simulink model "fftAnalysisSynthesis"  (R2022a)
settings: Solver=FixedStepDiscrete  StartTime=0.0  StopTime=simParams.stopTime  RelTol=1e-3
PostLoadFcn:
  | postLoadCallback
InitFcn:
  | initCallback
StopFcn:
  | stopCallback
values from neighbouring files (symbols this model uses):
  modelParams = createFFTFilters(modelParams)    [createModelParams.m]
libraries: hdlsllib x15, simulink x6, dspsrcs4 x3, dsphdlxfrm2 x2, dspsigops x1
CloseFcn:
  | closeCallback
settings Model: Creator=Ross  LastModifiedBy=Ross_admin
settings SolverCC: AlgebraicLoopSolver=TrustRegion
settings DataIOCC: ReturnWorkspaceOutputs=off
settings OptimizationCC: BlockReduction=off  ConditionallyExecuteInputs=off  DefaultParameterBehavior=Inlined
settings DebuggingCC: ReadBeforeWriteMsg=DisableAll  WriteAfterWriteMsg=DisableAll  WriteAfterReadMsg=DisableAll  AlgebraicLoopMsg=error  MultiTaskDSMMsg=none  SingleTaskRateTransMsg=error  UnconnectedInputMsg=warning  UnconnectedOutputMsg=warning  UnconnectedLineMsg=warning  PregeneratedLibrarySubsystemCodeDiagnostic=none  SFMachineParentedDataDiag=warning  ArithmeticOperatorsInVariantConditions=warning
settings HardwareCC: ProdBitPerPointer=32  ProdBitPerSizeT=32  ProdBitPerPtrDiffT=32  ProdLargestAtomicFloat=None  ProdIntDivRoundTo=Undefined  ProdEndianess=Unspecified  ProdWordSize=32  ProdHWDeviceType=ASIC/FPGA->ASIC/FPGA  TargetBitPerPointer=64  TargetBitPerSizeT=64  TargetBitPerPtrDiffT=64  TargetLongLongMode=on  TargetIntDivRoundTo=Zero  TargetEndianess=LittleEndian  TargetWordSize=64  TargetHWDeviceType=Custom Processor->MATLAB Host Computer  ProdEqTarget=off
settings ModelReferenceCC: UpdateModelReferenceTargets=IfOutOfDate
settings SFSimCC: SFSimEcho=off  SimUseLocalCustomCode=off  CustomCodeUndefinedFunction=UseInterfaceOnly
settings RTWCC: RTWUseLocalCustomCode=off  DLArmComputeVersion=19.05

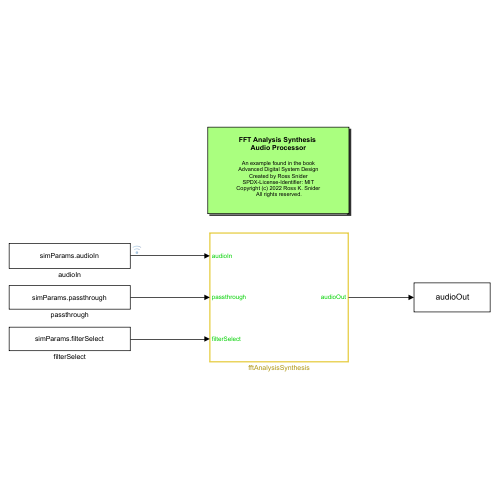
[thumbnail: Simulink's stored preview of the top-level diagram]
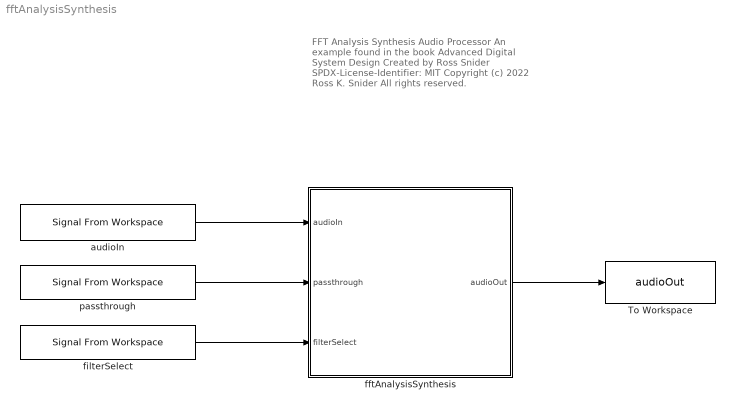
== system fftAnalysisSynthesis ==
  note: FFT Analysis Synthesis
      | Audio Processor
      |
      | An example found in the book
      | Advanced Digital System Design
      | Created by Ross Snider
      | SPDX-License-Identifier: MIT
      | Copyright (c) 2022 Ross K. Snider
      | All rights reserved.
  To Workspace : ToWorkspace  VariableName=audioOut  SampleTime=-1
      settings: Save2DSignal=2-D array (concatenate along first dimension)
  audioIn : dspsrcs4/Signal From Workspace  X=simParams.audioIn  Ts=modelParams.audio.samplePeriod  nsamps=1  OutputAfterFinalValue=Setting to zero  ignoreOrWarnInputAndFrameLengths=off  OutputFrames=off
  fftAnalysisSynthesis : Subsystem  TreatAsAtomicUnit=on
  filterSelect : dspsrcs4/Signal From Workspace  X=simParams.filterSelect  Ts=modelParams.audio.samplePeriod  nsamps=1  OutputAfterFinalValue=Holding final value  ignoreOrWarnInputAndFrameLengths=off  OutputFrames=off
  passthrough : dspsrcs4/Signal From Workspace  X=simParams.passthrough  Ts=modelParams.audio.samplePeriod  nsamps=1  OutputAfterFinalValue=Holding final value  ignoreOrWarnInputAndFrameLengths=off  OutputFrames=off
  wires:
  fftAnalysisSynthesis/1(audioOut) -> To Workspace/1
  audioIn/1 -> fftAnalysisSynthesis/1(audioIn)
  passthrough/1 -> fftAnalysisSynthesis/2(passthrough)
  filterSelect/1 -> fftAnalysisSynthesis/3(filterSelect)

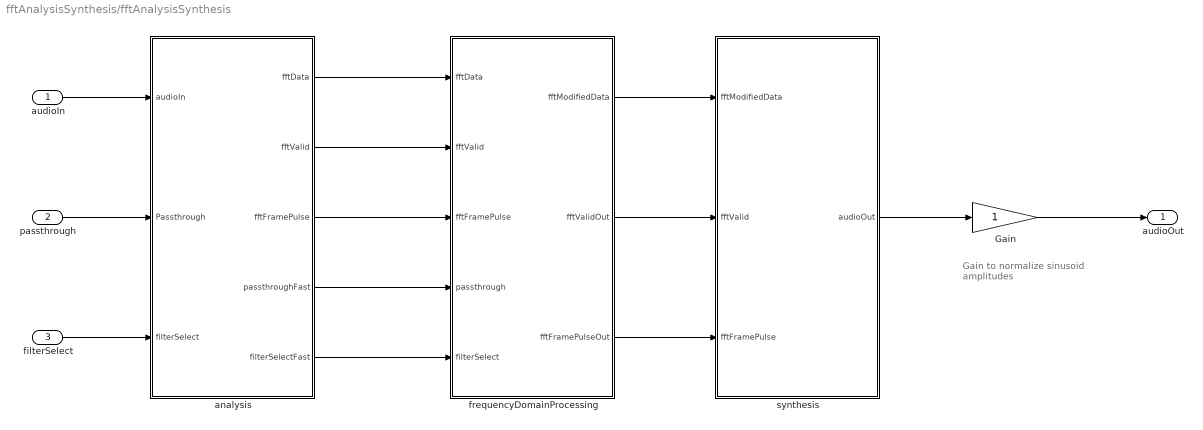
== system fftAnalysisSynthesis/fftAnalysisSynthesis ==
  note: Gain to normalize
      | sinusoid amplitudes
  audioIn : Inport
  passthrough : Inport  Port=2
  filterSelect : Inport  Port=3
  Gain : Gain  OutDataTypeStr=Inherit: Same as input  ParamDataTypeStr=Inherit: Same as input
  analysis : Subsystem
  frequencyDomainProcessing : Subsystem
  synthesis : Subsystem
  audioOut : Outport  VectorParamsAs1DForOutWhenUnconnected=off
  wires:
  audioIn/1 -> analysis/1(audioIn)
  synthesis/1(audioOut) -> Gain/1
  analysis/1(fftData) -> frequencyDomainProcessing/1(fftData)
  analysis/2(fftValid) -> frequencyDomainProcessing/2(fftValid)
  analysis/3(fftFramePulse) -> frequencyDomainProcessing/3(fftFramePulse)
  frequencyDomainProcessing/1(fftModifiedData) -> synthesis/1(fftModifiedData)
  frequencyDomainProcessing/2(fftValidOut) -> synthesis/2(fftValid)
  frequencyDomainProcessing/3(fftFramePulseOut) -> synthesis/3(fftFramePulse)
  analysis/4(passthroughFast) -> frequencyDomainProcessing/4(passthrough)
  passthrough/1 -> analysis/2(Passthrough)
  analysis/5(filterSelectFast) -> frequencyDomainProcessing/5(filterSelect)
  filterSelect/1 -> analysis/3(filterSelect)
  Gain/1 -> audioOut/1

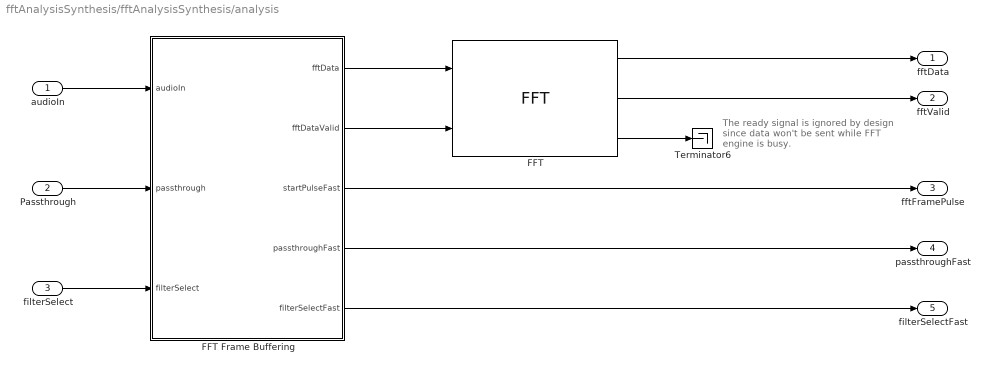
== system fftAnalysisSynthesis/fftAnalysisSynthesis/analysis ==
  note: The ready signal is ignored by design
      | since data won't be sent while FFT
      | engine is busy.
  audioIn : Inport
  Passthrough : Inport  Port=2
  filterSelect : Inport  Port=3
  FFT : dsphdlxfrm2/FFT  FFTLength=modelParams.fft.size  Architecture=Burst Radix 2  ComplexMultiplication=Use 4 multipliers and 2 adders  BitReversedOutput=off  BitReversedInput=off  Normalize=off  SimulateUsing=Code generation  RoundingMethod=Floor  ResetInputPort=off  StartOutputPort=off  EndOutputPort=off
      settings: SourceProductBaseCode=HS
  FFT Frame Buffering : Subsystem
  Terminator6 : Terminator
  fftData : Outport  VectorParamsAs1DForOutWhenUnconnected=off
  fftValid : Outport  Port=2  VectorParamsAs1DForOutWhenUnconnected=off
  fftFramePulse : Outport  Port=3  VectorParamsAs1DForOutWhenUnconnected=off
  passthroughFast : Outport  Port=4
  filterSelectFast : Outport  Port=5
  wires:
  FFT/3 -> Terminator6/1
  FFT Frame Buffering/3(startPulseFast) -> fftFramePulse/1
  audioIn/1 -> FFT Frame Buffering/1(audioIn)
  FFT Frame Buffering/2(fftDataValid) -> FFT/2
  FFT Frame Buffering/1(fftData) -> FFT/1
  FFT/1 -> fftData/1
  FFT/2 -> fftValid/1
  FFT Frame Buffering/4(passthroughFast) -> passthroughFast/1
  Passthrough/1 -> FFT Frame Buffering/2(passthrough)
  filterSelect/1 -> FFT Frame Buffering/3(filterSelect)
  FFT Frame Buffering/5(filterSelectFast) -> filterSelectFast/1

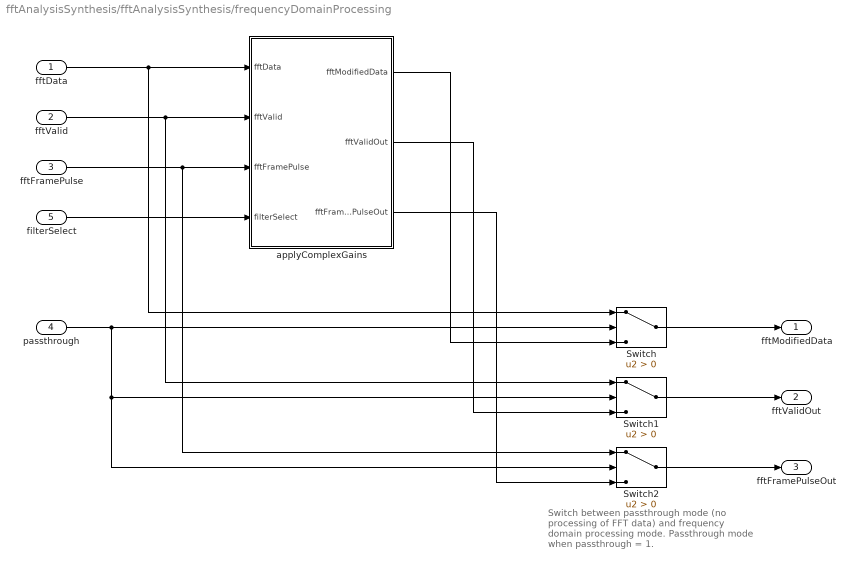
== system fftAnalysisSynthesis/fftAnalysisSynthesis/frequencyDomainProcessing ==
  note: Switch between passthrough mode
      | (no processing of FFT data)
      | and frequency domain processing mode.
      | Passthrough mode when passthrough = 1.
  fftData : Inport
  fftValid : Inport  Port=2
  fftFramePulse : Inport  Port=3
  passthrough : Inport  Port=4
  filterSelect : Inport  Port=5
  Switch : Switch  Criteria=u2 > Threshold  SaturateOnIntegerOverflow=off  InputSameDT=off
  Switch1 : Switch  Criteria=u2 > Threshold  SaturateOnIntegerOverflow=off  InputSameDT=off
  Switch2 : Switch  Criteria=u2 > Threshold  SaturateOnIntegerOverflow=off  InputSameDT=off
  applyComplexGains : Subsystem
  fftModifiedData : Outport  VectorParamsAs1DForOutWhenUnconnected=off
  fftValidOut : Outport  Port=2  VectorParamsAs1DForOutWhenUnconnected=off
  fftFramePulseOut : Outport  Port=3
  wires:
  fftData/1 -> applyComplexGains/1(fftData), Switch/1
  fftValid/1 -> applyComplexGains/2(fftValid), Switch1/1
  applyComplexGains/1(fftModifiedData) -> Switch/3
  applyComplexGains/2(fftValidOut) -> Switch1/3
  fftFramePulse/1 -> applyComplexGains/3(fftFramePulse), Switch2/1
  passthrough/1 -> Switch2/2, Switch1/2, Switch/2
  Switch/1 -> fftModifiedData/1
  applyComplexGains/3(fftFramePulseOut) -> Switch2/3
  Switch1/1 -> fftValidOut/1
  Switch2/1 -> fftFramePulseOut/1
  filterSelect/1 -> applyComplexGains/4(filterSelect)

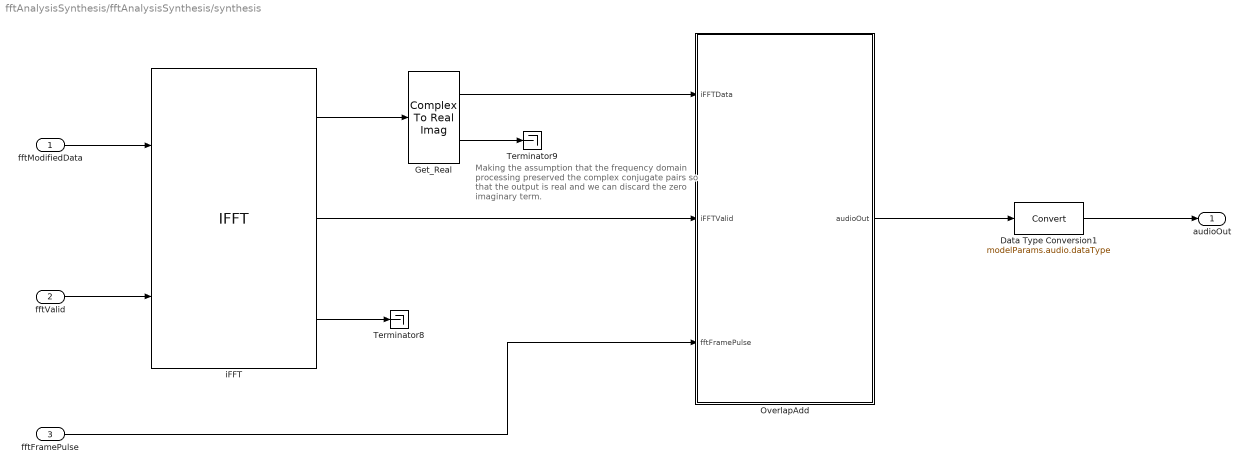
== system fftAnalysisSynthesis/fftAnalysisSynthesis/synthesis ==
  note: Making the assumption that the frequency domain processing preserved the complex conjugate pairs so that the output is real and we can discard the zero imaginary term.
  fftModifiedData : Inport
  fftValid : Inport  Port=2
  fftFramePulse : Inport  Port=3
  Data Type Conversion1 : DataTypeConversion  OutDataTypeStr=modelParams.audio.dataType  SaturateOnIntegerOverflow=off  RndMeth=Floor
  Get_Real : ComplexToRealImag
  OverlapAdd : Subsystem
  Terminator8 : Terminator
  Terminator9 : Terminator
  iFFT : dsphdlxfrm2/IFFT  FFTLength=modelParams.fft.size  Architecture=Burst Radix 2  ComplexMultiplication=Use 4 multipliers and 2 adders  BitReversedOutput=off  BitReversedInput=off  Normalize=on  SimulateUsing=Code generation  RoundingMethod=Floor  ResetInputPort=off  StartOutputPort=off  EndOutputPort=off
      settings: SourceProductBaseCode=HS
  audioOut : Outport  VectorParamsAs1DForOutWhenUnconnected=off
  wires:
  iFFT/3 -> Terminator8/1
  iFFT/2 -> OverlapAdd/2(iFFTValid)
  Get_Real/1 -> OverlapAdd/1(iFFTData)
  fftModifiedData/1 -> iFFT/1
  Data Type Conversion1/1 -> audioOut/1
  iFFT/1 -> Get_Real/1
  Get_Real/2 -> Terminator9/1
  fftValid/1 -> iFFT/2
  fftFramePulse/1 -> OverlapAdd/3(fftFramePulse)
  OverlapAdd/1(audioOut) -> Data Type Conversion1/1

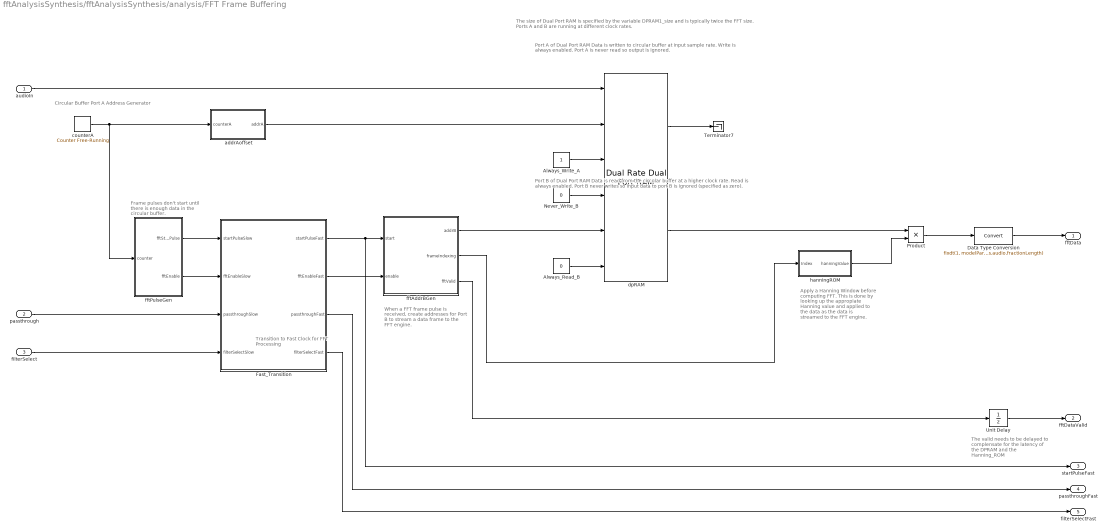
== system fftAnalysisSynthesis/fftAnalysisSynthesis/analysis/FFT Frame Buffering ==
  note: The valid needs to be delayed
      | to complensate for the latency
      | of the DPRAM and the
      | Hanning_ROM
  note: When a FFT frame pulse
      | is received, create addresses for
      | Port B to stream a data frame
      | to the FFT engine.
  note: Apply a Hanning Window
      | before computing FFT.  This
      | is done by looking up the
      | appropiate Hanning value
      | and applied to the data as the
      | data is streamed to the
      | FFT engine.
  note: Frame pulses don't start
      | until there is enough data
      | in the circular buffer.
  note: The size of Dual Port RAM is specified by the variable DPRAM1_size
      | and is typically twice the FFT size.  Ports A and B are running at different clock rates.
  note: Circular Buffer
      | Port A Address Generator
  note: Port A of Dual Port RAM
      |
      | Data is written to circular buffer at input sample rate.
      | Write is always enabled.  Port A is never read so output is ignored.
  note: Transition to
      | Fast Clock
      | for FFT Processing
  note: Port B of Dual Port RAM
      |
      | Data is read from the circular buffer at a higher clock rate.
      | Read is always enabled.  Port B never writes so input data to port B
      | is ignored (specified as zero).
  audioIn : Inport
  passthrough : Inport  Port=2
  filterSelect : Inport  Port=3
  Always_Read_B : Constant  Value=0  OutDataTypeStr=boolean  SampleTime=modelParams.audio.samplePeriod/modelParams.system.upsample_Factor
  Always_Write_A : Constant  OutDataTypeStr=boolean  SampleTime=modelParams.audio.samplePeriod
  Data Type Conversion : DataTypeConversion  OutDataTypeStr=fixdt(1, modelParams.audio.wordLength, modelParams.audio.fractionLength)  SaturateOnIntegerOverflow=off  RndMeth=Floor
  Fast_Transition : Subsystem
  Never_Write_B : Constant  Value=0  OutDataTypeStr=modelParams.audio.dataType  SampleTime=modelParams.audio.samplePeriod/modelParams.system.upsample_Factor
  Product : Product
  Terminator7 : Terminator
  Unit Delay : UnitDelay  SampleTime=-1  HasFrameUpgradeWarning=on
  addrAoffset : Subsystem
  counterA : simulink/Sources/Counter Free-Running  NumBits=modelParams.dpram1.address_size  tsamp=modelParams.audio.samplePeriod
  dpRAM : hdlsllib/HDL RAMs/Dual Rate Dual Port RAM  ram_size=modelParams.dpram1.address_size
      settings: SourceProductBaseCode=SL
  fftAddrBGen : Subsystem
  fftPulseGen : Subsystem
  hanningROM : Subsystem
  fftData : Outport  VectorParamsAs1DForOutWhenUnconnected=off
  fftDataValid : Outport  Port=2  VectorParamsAs1DForOutWhenUnconnected=off
  startPulseFast : Outport  Port=3  VectorParamsAs1DForOutWhenUnconnected=off
  passthroughFast : Outport  Port=4
  filterSelectFast : Outport  Port=5
  wires:
  Always_Write_A/1 -> dpRAM/3
  Never_Write_B/1 -> dpRAM/4
  Always_Read_B/1 -> dpRAM/6
  dpRAM/1 -> Terminator7/1
  fftAddrBGen/3(fftValid) -> Unit Delay/1
  fftAddrBGen/1(addrB) -> dpRAM/5
  counterA/1 -> addrAoffset/1(counterA), fftPulseGen/1(counter)
  audioIn/1 -> dpRAM/1
  addrAoffset/1(addrA) -> dpRAM/2
  fftAddrBGen/2(frameIndexing) -> hanningROM/1(Index)
  Product/1 -> Data Type Conversion/1
  dpRAM/2 -> Product/1
  hanningROM/1(hanningValue) -> Product/2
  Data Type Conversion/1 -> fftData/1
  Fast_Transition/1(startPulseFast) -> startPulseFast/1, fftAddrBGen/1(start)
  fftPulseGen/1(fftStartPulse) -> Fast_Transition/1(startPulseSlow)
  fftPulseGen/2(fftEnable) -> Fast_Transition/2(fftEnableSlow)
  Fast_Transition/2(fftEnableFast) -> fftAddrBGen/2(enable)
  Unit Delay/1 -> fftDataValid/1
  passthrough/1 -> Fast_Transition/3(passthroughSlow)
  Fast_Transition/3(passthroughFast) -> passthroughFast/1
  filterSelect/1 -> Fast_Transition/4(filterSelectSlow)
  Fast_Transition/4(filterSelectFast) -> filterSelectFast/1

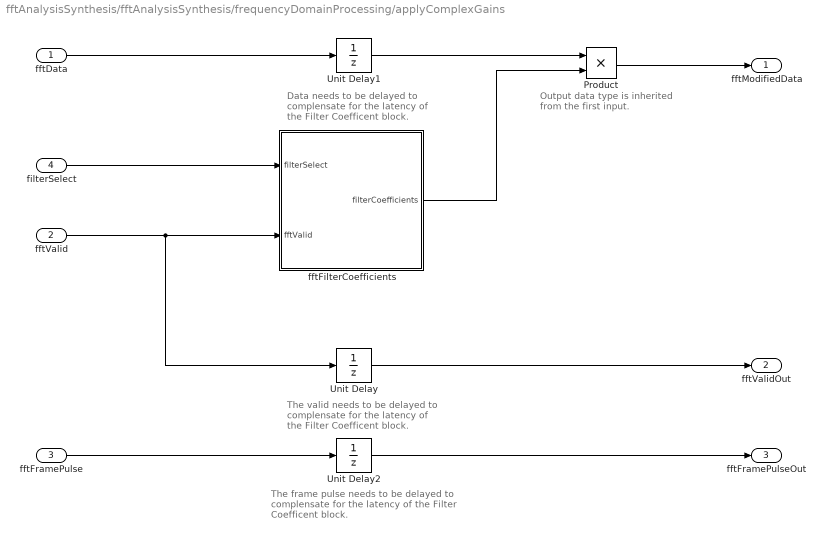
== system fftAnalysisSynthesis/fftAnalysisSynthesis/frequencyDomainProcessing/applyComplexGains ==
  note: Output data type is inherited
      | from the first input.
  note: The frame pulse needs to be delayed
      | to complensate for the latency
      | of the Filter Coefficent block.
  note: The valid needs to be delayed
      | to complensate for the latency
      | of the Filter Coefficent block.
  note: Data needs to be delayed
      | to complensate for the latency
      | of the Filter Coefficent block.
  fftData : Inport
  fftValid : Inport  Port=2
  fftFramePulse : Inport  Port=3
  filterSelect : Inport  Port=4
  Product : Product  OutDataTypeStr=Inherit: Same as first input
  Unit Delay : UnitDelay  SampleTime=-1  HasFrameUpgradeWarning=on
  Unit Delay1 : UnitDelay  SampleTime=-1  HasFrameUpgradeWarning=on
  Unit Delay2 : UnitDelay  SampleTime=-1  HasFrameUpgradeWarning=on
  fftFilterCoefficients : Subsystem
  fftModifiedData : Outport
  fftValidOut : Outport  Port=2
  fftFramePulseOut : Outport  Port=3
  wires:
  fftValid/1 -> Unit Delay/1, fftFilterCoefficients/2(fftValid)
  fftData/1 -> Unit Delay1/1
  fftFramePulse/1 -> Unit Delay2/1
  Unit Delay2/1 -> fftFramePulseOut/1
  filterSelect/1 -> fftFilterCoefficients/1(filterSelect)
  fftFilterCoefficients/1(filterCoefficients) -> Product/2
  Product/1 -> fftModifiedData/1
  Unit Delay/1 -> fftValidOut/1
  Unit Delay1/1 -> Product/1

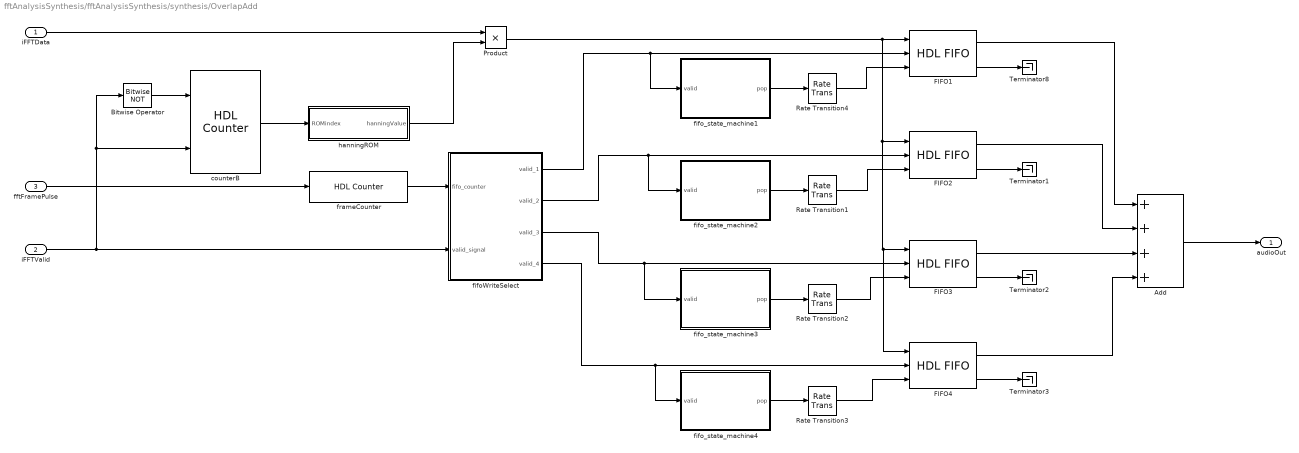
== system fftAnalysisSynthesis/fftAnalysisSynthesis/synthesis/OverlapAdd ==
  iFFTData : Inport
  iFFTValid : Inport  Port=2
  fftFramePulse : Inport  Port=3
  Add : Sum  Inputs=4
  Bitwise Operator : simulink/Logic and Bit Operations/Bitwise Operator  logicop=NOT  UseBitMask=off  BitMask=bin2dec('11011001')  BitMaskRealWorld=Stored Integer
  FIFO{1..4} (4 alike) : hdlsllib/HDL RAMs/HDL FIFO  fifo_size=modelParams.fft.size  mode=Classic  ratio=modelParams.system.upsample_Factor  push_msg=Warning  pop_msg=Warning  show_empty=off  show_full=on  show_num=off  LabelModeActiveChoice_Mode=Classic  rst_port=off
      settings: SourceProductBaseCode=SL
  Product : Product  OutDataTypeStr=Inherit: Same as first input
  Rate Transition{1..4} (4 alike) : RateTransition  OutPortSampleTimeOpt=Multiple of input port sample time  OutPortSampleTimeMultiple=modelParams.system.upsample_Factor
  Terminator{1..3,8} (4 alike) : Terminator
  counterB : hdlsllib/Sources/HDL Counter  CountType=Count limited  CountInit=0  CountStep=1  CountMax=modelParams.fft.size  CountFromType=Initial value  CountFrom=0  CountResetPort=on  CountLoadPort=off  CountEnbPort=on  CountDirPort=off  CountHitOutputPort=off  CountDataType=Unsigned  CountWordLen=modelParams.dpram1.address_size  CountFracLen=0  CountSampTime=1
  fifoWriteSelect : MATLAB Function  TreatAsAtomicUnit=on
  fifo_state_machine1 : MATLAB Function  TreatAsAtomicUnit=on
  fifo_state_machine2 : MATLAB Function  TreatAsAtomicUnit=on
  fifo_state_machine3 : MATLAB Function  TreatAsAtomicUnit=on
  fifo_state_machine4 : MATLAB Function  TreatAsAtomicUnit=on
  frameCounter : hdlsllib/Sources/HDL Counter  CountType=Free running  CountInit=2  CountStep=1  CountMax=1024  CountFromType=Initial value  CountFrom=2  CountResetPort=off  CountLoadPort=off  CountEnbPort=on  CountDirPort=off  CountHitOutputPort=off  CountDataType=Unsigned  CountWordLen=2  CountFracLen=0  CountSampTime=1
  hanningROM : Subsystem
  audioOut : Outport  VectorParamsAs1DForOutWhenUnconnected=off
  wires:
  FIFO1/1 -> Add/1
  FIFO3/1 -> Add/3
  fftFramePulse/1 -> frameCounter/1
  FIFO2/1 -> Add/2
  fifoWriteSelect/3(valid_3) -> fifo_state_machine3/1(valid), FIFO3/2
  fifoWriteSelect/4(valid_4) -> fifo_state_machine4/1(valid), FIFO4/2
  FIFO4/1 -> Add/4
  fifoWriteSelect/1(valid_1) -> fifo_state_machine1/1(valid), FIFO1/2
  fifoWriteSelect/2(valid_2) -> fifo_state_machine2/1(valid), FIFO2/2
  Add/1 -> audioOut/1
  frameCounter/1 -> fifoWriteSelect/1(fifo_counter)
  FIFO4/2 -> Terminator3/1
  FIFO2/2 -> Terminator1/1
  FIFO3/2 -> Terminator2/1
  Bitwise Operator/1 -> counterB/1
  iFFTValid/1 -> counterB/2, Bitwise Operator/1, fifoWriteSelect/2(valid_signal)
  iFFTData/1 -> Product/1
  hanningROM/1(hanningValue) -> Product/2
  counterB/1 -> hanningROM/1(ROMindex)
  fifo_state_machine1/1(pop) -> Rate Transition4/1
  Rate Transition4/1 -> FIFO1/3
  FIFO1/2 -> Terminator8/1
  fifo_state_machine2/1(pop) -> Rate Transition1/1
  Rate Transition1/1 -> FIFO2/3
  fifo_state_machine3/1(pop) -> Rate Transition2/1
  Rate Transition2/1 -> FIFO3/3
  fifo_state_machine4/1(pop) -> Rate Transition3/1
  Rate Transition3/1 -> FIFO4/3
  Product/1 -> FIFO4/1, FIFO3/1, FIFO2/1, FIFO1/1

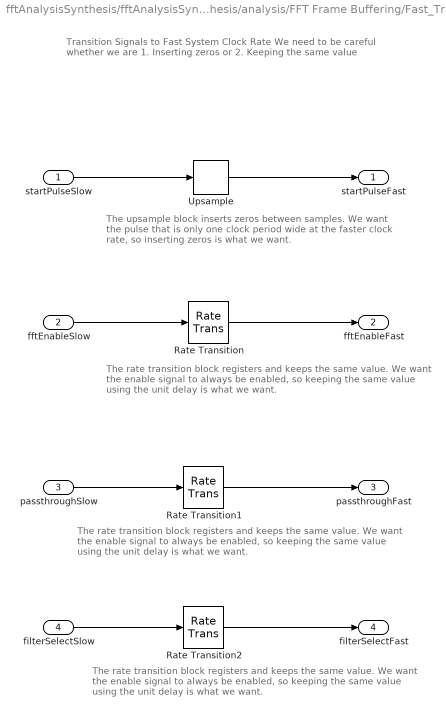
== system fftAnalysisSynthesis/fftAnalysisSynthesis/analysis/FFT Frame Buffering/Fast_Transition ==
  note: The upsample block inserts zeros between samples.
      | We want the pulse that is only one clock period wide at the
      | faster clock rate, so inserting zeros is what we want.
  note: The rate transition block registers and keeps the same
      | value. We want the enable signal to always be enabled,
      | so keeping the same value using the unit delay is what we want.
  note: The rate transition block registers and keeps the same
      | value. We want the enable signal to always be enabled,
      | so keeping the same value using the unit delay is what we want.
  note: The rate transition block registers and keeps the same
      | value. We want the enable signal to always be enabled,
      | so keeping the same value using the unit delay is what we want.
  note: Transition Signals to Fast System Clock Rate
      | We need to be careful whether we are
      | 1. Inserting zeros
      | or
      | 2. Keeping the same value
  startPulseSlow : Inport
  fftEnableSlow : Inport  Port=2
  passthroughSlow : Inport  Port=3
  filterSelectSlow : Inport  Port=4
  Rate Transition : RateTransition  OutPortSampleTimeOpt=Multiple of input port sample time  OutPortSampleTimeMultiple=1/modelParams.system.upsample_Factor
  Rate Transition1 : RateTransition  OutPortSampleTimeOpt=Multiple of input port sample time  OutPortSampleTimeMultiple=1/modelParams.system.upsample_Factor
  Rate Transition2 : RateTransition  InitialCondition=3  OutPortSampleTimeOpt=Multiple of input port sample time  OutPortSampleTimeMultiple=1/modelParams.system.upsample_Factor
  Upsample : dspsigops/Upsample  N=modelParams.system.upsample_Factor  phase=0  RateOptions=Allow multirate processing  ic=0  mode=Unused parameter value
  startPulseFast : Outport
  fftEnableFast : Outport  Port=2
  passthroughFast : Outport  Port=3
  filterSelectFast : Outport  Port=4
  wires:
  startPulseSlow/1 -> Upsample/1
  Rate Transition/1 -> fftEnableFast/1
  fftEnableSlow/1 -> Rate Transition/1
  Upsample/1 -> startPulseFast/1
  passthroughSlow/1 -> Rate Transition1/1
  Rate Transition1/1 -> passthroughFast/1
  filterSelectSlow/1 -> Rate Transition2/1
  Rate Transition2/1 -> filterSelectFast/1

== system fftAnalysisSynthesis/fftAnalysisSynthesis/analysis/FFT Frame Buffering/addrAoffset ==
  note: Adding 1 to counter since the read pointer (addr_B) can catch the write pointer (addr_A)
      | if SysRate_Upsample_Factor is large enough and Simulink will throw an error.
      | It would be nice if the HDL Coder allowed a read-before-write option when
      | the addresses are identical, which some memories support.
  counterA : Inport
  Add : Sum  OutDataTypeStr=fixdt(0,modelParams.dpram1.address_size,0)
  writeOffset : Constant  OutDataTypeStr=fixdt(0,modelParams.dpram1.address_size,0)  SampleTime=modelParams.audio.samplePeriod
  addrA : Outport  VectorParamsAs1DForOutWhenUnconnected=off
  wires:
  writeOffset/1 -> Add/2
  Add/1 -> addrA/1
  counterA/1 -> Add/1

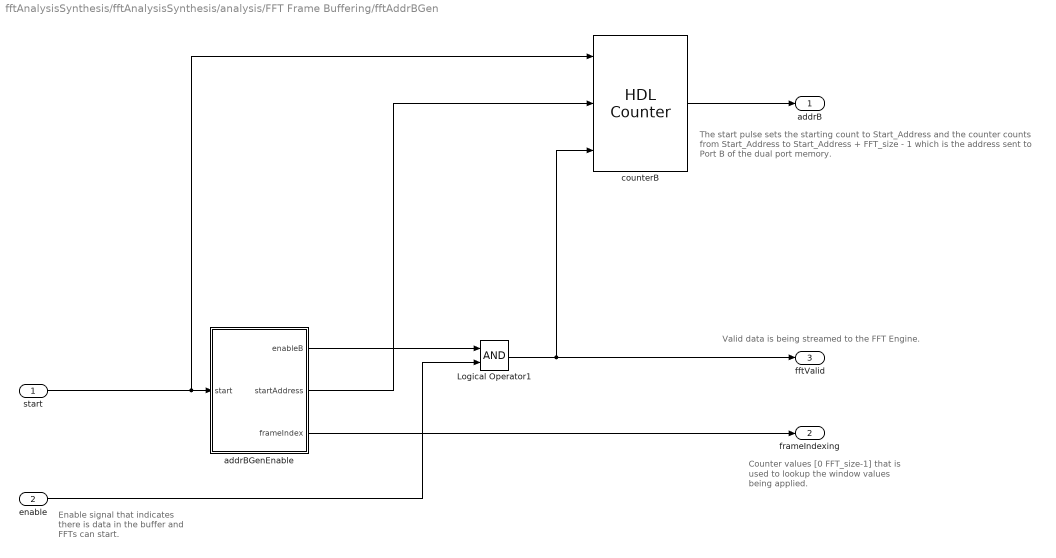
== system fftAnalysisSynthesis/fftAnalysisSynthesis/analysis/FFT Frame Buffering/fftAddrBGen ==
  note: Counter values [0 FFT_size-1] that
      | is used to lookup the window values
      | being applied.
  note: Valid data is being streamed to the FFT Engine.
  note: Enable signal that indicates
      | there is data in the buffer
      | and FFTs can start.
  note: The start pulse sets the starting count to Start_Address
      |  and the counter counts from Start_Address to Start_Address + FFT_size - 1
      | which is the address sent to Port B of the dual port memory.
  start : Inport
  enable : Inport  Port=2
  Logical Operator1 : Logic  AllPortsSameDT=off  OutDataTypeStr=boolean
  addrBGenEnable : Subsystem
  counterB : hdlsllib/Sources/HDL Counter  CountType=Free running  CountInit=modelParams.dpram1.init  CountStep=1  CountMax=1024  CountFromType=Initial value  CountFrom=modelParams.dpram1.init  CountResetPort=off  CountLoadPort=on  CountEnbPort=on  CountDirPort=off  CountHitOutputPort=off  CountDataType=Unsigned  CountWordLen=modelParams.dpram1.address_size  CountFracLen=0  CountSampTime=1
  addrB : Outport  VectorParamsAs1DForOutWhenUnconnected=off
  frameIndexing : Outport  Port=2  VectorParamsAs1DForOutWhenUnconnected=off
  fftValid : Outport  Port=3  VectorParamsAs1DForOutWhenUnconnected=off
  wires:
  counterB/1 -> addrB/1
  start/1 -> counterB/1, addrBGenEnable/1(start)
  addrBGenEnable/1(enableB) -> Logical Operator1/1
  addrBGenEnable/2(startAddress) -> counterB/2
  enable/1 -> Logical Operator1/2
  addrBGenEnable/3(frameIndex) -> frameIndexing/1
  Logical Operator1/1 -> counterB/3, fftValid/1

== system fftAnalysisSynthesis/fftAnalysisSynthesis/analysis/FFT Frame Buffering/fftPulseGen ==
  note: Don't send out FFT frame start pulses
      | until circular buffer has filled.
  counter : Inport
  fftFramePulseGen : Subsystem
  waitForData : Subsystem
  fftStartPulse : Outport  VectorParamsAs1DForOutWhenUnconnected=off
  fftEnable : Outport  Port=2  VectorParamsAs1DForOutWhenUnconnected=off
  wires:
  counter/1 -> fftFramePulseGen/1("counterValue ")
  waitForData/1(fftFramePulse) -> fftStartPulse/1
  waitForData/2(enableFFTframes) -> fftEnable/1
  fftFramePulseGen/1(framePulse) -> waitForData/1(framePulse)

== system fftAnalysisSynthesis/fftAnalysisSynthesis/analysis/FFT Frame Buffering/hanningROM ==
  Index : Inport
  Lookup Table : Lookup_n-D  NumberOfTableDimensions=1  BreakpointsForDimension1=[0:modelParams.fft.size-1]  IndexSearchMethod=Evenly spaced points  Table=hanning(modelParams.fft.size)  InterpMethod=Flat  ExtrapMethod=Clip  DiagnosticForOutOfRangeInput=Warning  UseLastTableValue=on  OutDataTypeStr=fixdt(1,24,23)  RndMeth=Simplest
  Unit Delay : UnitDelay  SampleTime=-1  HasFrameUpgradeWarning=on
  hanningValue : Outport  VectorParamsAs1DForOutWhenUnconnected=off
  wires:
  Unit Delay/1 -> hanningValue/1
  Index/1 -> Lookup Table/1
  Lookup Table/1 -> Unit Delay/1

== system fftAnalysisSynthesis/fftAnalysisSynthesis/frequencyDomainProcessing/applyComplexGains/fftFilterCoefficients ==
  filterSelect : Inport
  fftValid : Inport  Port=2
  fftROMindexing : Subsystem
  filterChoice : Subsystem
  filterCoefficients : Outport
  wires:
  fftROMindexing/1(ROMindex) -> filterChoice/2(ROMindex)
  fftValid/1 -> fftROMindexing/1(fftValid)
  filterSelect/1 -> filterChoice/1(filterSelect)
  filterChoice/1(filterCoefficients) -> filterCoefficients/1

== system fftAnalysisSynthesis/fftAnalysisSynthesis/synthesis/OverlapAdd/hanningROM ==
  ROMindex : Inport
  Bit Slice : hdlsllib/Logic and Bit Operations/Bit Slice  lidx=modelParams.fft.Nbits - 1  ridx=0
      settings: SourceProductBaseCode=SL
  Lookup Table : Lookup_n-D  NumberOfTableDimensions=1  BreakpointsForDimension1=[0:modelParams.fft.size-1]  IndexSearchMethod=Evenly spaced points  Table=hanning(modelParams.fft.size)  InterpMethod=Flat  ExtrapMethod=Clip  DiagnosticForOutOfRangeInput=Error  UseLastTableValue=on  OutDataTypeStr=fixdt(1,24,22)  RndMeth=Simplest
  Unit Delay : UnitDelay  SampleTime=-1  HasFrameUpgradeWarning=on
  hanningValue : Outport  VectorParamsAs1DForOutWhenUnconnected=off
  wires:
  Unit Delay/1 -> hanningValue/1
  ROMindex/1 -> Bit Slice/1
  Lookup Table/1 -> Unit Delay/1
  Bit Slice/1 -> Lookup Table/1

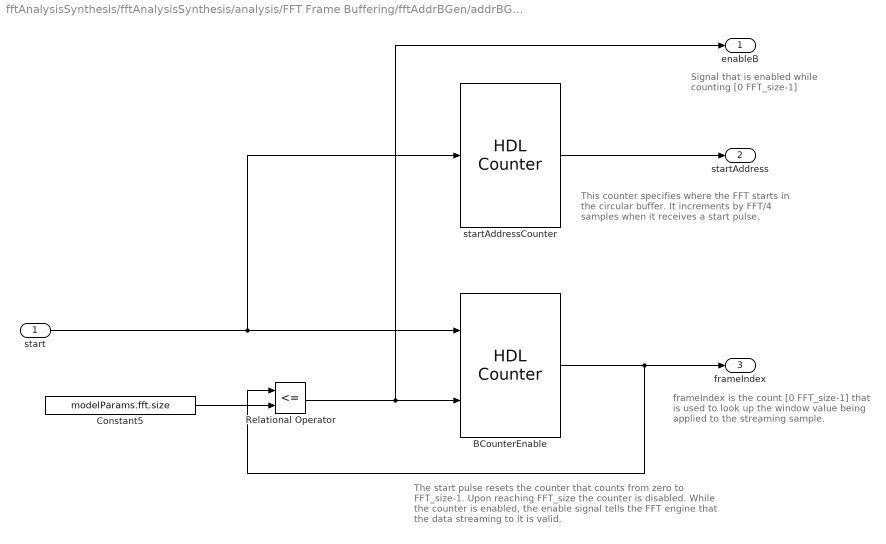
== system fftAnalysisSynthesis/fftAnalysisSynthesis/analysis/FFT Frame Buffering/fftAddrBGen/addrBGenEnable ==
  note: Signal that is enabled while
      | counting [0 FFT_size-1]
  note: frameIndex is the count [0 FFT_size-1]
      | that is used to look up the window value
      | being applied to the streaming sample.
  note: This counter specifies where the FFT starts
      | in the circular buffer.  It increments by FFT/4
      | samples when it receives a start pulse.
  note: The start pulse resets the counter that counts
      | from zero to FFT_size-1.  Upon reaching FFT_size
      | the counter is disabled.  While the counter is enabled,
      | the enable signal tells the FFT engine that the data streaming
      | to it is valid.
  start : Inport
  BCounterEnable : hdlsllib/Sources/HDL Counter  CountType=Count limited  CountInit=0  CountStep=1  CountMax=modelParams.fft.size  CountFromType=Specify  CountFrom=0  CountResetPort=on  CountLoadPort=off  CountEnbPort=on  CountDirPort=off  CountHitOutputPort=off  CountDataType=Unsigned  CountWordLen=modelParams.dpram1.address_size  CountFracLen=0  CountSampTime=1
  Constant5 : Constant  Value=modelParams.fft.size  OutDataTypeStr=fixdt(0,modelParams.fft.Nbits,0)  SampleTime=modelParams.audio.samplePeriod/modelParams.system.upsample_Factor
  Relational Operator : RelationalOperator  Operator=<=  OutDataTypeStr=boolean  ZeroCross=off  InputSameDT=off
  startAddressCounter : hdlsllib/Sources/HDL Counter  CountType=Free running  CountInit=0  CountStep=modelParams.fft.frame_shift  CountMax=25  CountFromType=Initial value  CountFrom=0  CountResetPort=off  CountLoadPort=off  CountEnbPort=on  CountDirPort=off  CountHitOutputPort=off  CountDataType=Unsigned  CountWordLen=modelParams.dpram1.address_size  CountFracLen=0  CountSampTime=1
  enableB : Outport  VectorParamsAs1DForOutWhenUnconnected=off
  startAddress : Outport  Port=2  VectorParamsAs1DForOutWhenUnconnected=off
  frameIndex : Outport  Port=3  VectorParamsAs1DForOutWhenUnconnected=off
  wires:
  Relational Operator/1 -> enableB/1, BCounterEnable/2
  Constant5/1 -> Relational Operator/2
  BCounterEnable/1 -> frameIndex/1, Relational Operator/1
  start/1 -> BCounterEnable/1, startAddressCounter/1
  startAddressCounter/1 -> startAddress/1

== system fftAnalysisSynthesis/fftAnalysisSynthesis/analysis/FFT Frame Buffering/fftPulseGen/fftFramePulseGen ==
  note: Create a FFT frame pulse that happens every FFT_size/4 samples.
      | We do this by watching when an appropriate subset of the counter bits
      | become zero.
  "counterValue " : Inport
  Bit Slice : hdlsllib/Logic and Bit Operations/Bit Slice  lidx=modelParams.fft.frame_shift_Nbits-1  ridx=0
      settings: SourceProductBaseCode=SL
  Compare To Zero : simulink/Logic and Bit Operations/Compare To Zero  relop===  OutDataTypeStr=boolean
  framePulse : Outport  VectorParamsAs1DForOutWhenUnconnected=off
  wires:
  "counterValue "/1 -> Bit Slice/1
  Compare To Zero/1 -> framePulse/1
  Bit Slice/1 -> Compare To Zero/1

== system fftAnalysisSynthesis/fftAnalysisSynthesis/analysis/FFT Frame Buffering/fftPulseGen/waitForData ==
  note: Frame pulses don't start
      | coming through until
      | circular buffer has data.
  note: Counter starts a zero and counts number of frame pulses.
      | Counter remains enabled while frame count is less than 4.
      | As soon as the counter reaches 4, it is disabled, which then
      | enables the frame pulses to pass through.
  note: framePulse
      | will pass through
      | when enabled
  note: Number of Frames
      | to wait before starting
  note: Start performing FFTs after enough data has filled the circular buffer.
      | This is due to the fact that we don't want the read pointer (addrB)
      | to catch up with the write pointer (addrA) because if it does,
      | the dpRAM will throw an assertion error.
  note: Enable signal that that indicates
      | that FFTs can start since there is
      | data in the buffer.
  framePulse : Inport
  Bitwise Operator : simulink/Logic and Bit Operations/Bitwise Operator  logicop=NOT  UseBitMask=off  BitMask=bin2dec('11011001')  BitMaskRealWorld=Stored Integer
  Compare To Constant : simulink/Logic and Bit Operations/Compare To Constant  relop=<  const=4  OutDataTypeStr=boolean
  Logical Operator : Logic  AllPortsSameDT=off  OutDataTypeStr=boolean
  Logical Operator1 : Logic  AllPortsSameDT=off  OutDataTypeStr=boolean
  initialFrameCount : hdlsllib/Sources/HDL Counter  CountType=Count limited  CountInit=0  CountStep=1  CountMax=4  CountFromType=Specify  CountFrom=0  CountResetPort=off  CountLoadPort=off  CountEnbPort=on  CountDirPort=off  CountHitOutputPort=off  CountDataType=Unsigned  CountWordLen=5  CountFracLen=0  CountSampTime=1
  fftFramePulse : Outport  VectorParamsAs1DForOutWhenUnconnected=off
  enableFFTframes : Outport  Port=2  VectorParamsAs1DForOutWhenUnconnected=off
  wires:
  Logical Operator1/1 -> fftFramePulse/1
  framePulse/1 -> Logical Operator/2, Logical Operator1/1
  initialFrameCount/1 -> Compare To Constant/1
  Logical Operator/1 -> initialFrameCount/1
  Compare To Constant/1 -> Bitwise Operator/1, Logical Operator/1
  Bitwise Operator/1 -> enableFFTframes/1, Logical Operator1/2

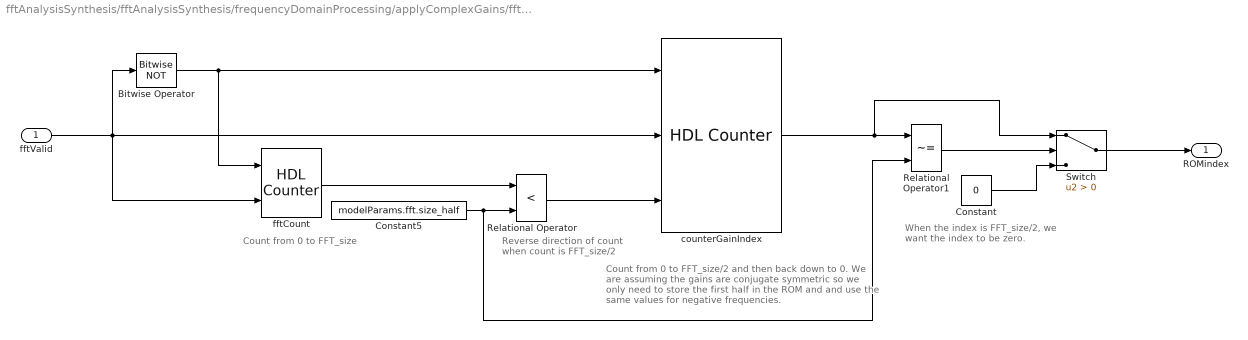
== system fftAnalysisSynthesis/fftAnalysisSynthesis/frequencyDomainProcessing/applyComplexGains/fftFilterCoefficients/fftROMindexing ==
  note: When the index is FFT_size/2,
      | we want the index to be zero.
  note: Count from 0 to FFT_size
  note: Reverse direction of
      | count when count
      | is FFT_size/2
  note: Count from 0 to FFT_size/2 and then back down to 0.
      | We are assuming the gains are conjugate symmetric
      | so we only need to store the first half in the ROM
      | and and use the same values for negative frequencies.
  fftValid : Inport
  Bitwise Operator : simulink/Logic and Bit Operations/Bitwise Operator  logicop=NOT  UseBitMask=off  BitMask=bin2dec('11011001')  BitMaskRealWorld=Stored Integer
  Constant : Constant  Value=0  OutDataTypeStr=fixdt(0,modelParams.fft.Nbits,0)  SampleTime=modelParams.audio.samplePeriod/modelParams.system.upsample_Factor
  Constant5 : Constant  Value=modelParams.fft.size_half  OutDataTypeStr=fixdt(0,modelParams.fft.Nbits,0)  SampleTime=modelParams.audio.samplePeriod/modelParams.system.upsample_Factor
  Relational Operator : RelationalOperator  Operator=<  OutDataTypeStr=boolean  ZeroCross=off  InputSameDT=off
  Relational Operator1 : RelationalOperator  Operator=~=  OutDataTypeStr=boolean  ZeroCross=off  InputSameDT=off
  Switch : Switch  Criteria=u2 > Threshold  SaturateOnIntegerOverflow=off  InputSameDT=off
  counterGainIndex : hdlsllib/Sources/HDL Counter  CountType=Free running  CountInit=0  CountStep=1  CountMax=25  CountFromType=Initial value  CountFrom=0  CountResetPort=on  CountLoadPort=off  CountEnbPort=on  CountDirPort=on  CountHitOutputPort=off  CountDataType=Unsigned  CountWordLen=modelParams.fft.Nbits  CountFracLen=0  CountSampTime=1
  fftCount : hdlsllib/Sources/HDL Counter  CountType=Free running  CountInit=0  CountStep=1  CountMax=25  CountFromType=Initial value  CountFrom=0  CountResetPort=on  CountLoadPort=off  CountEnbPort=on  CountDirPort=off  CountHitOutputPort=off  CountDataType=Unsigned  CountWordLen=modelParams.fft.Nbits  CountFracLen=0  CountSampTime=1
  ROMindex : Outport
  wires:
  Relational Operator/1 -> counterGainIndex/3
  Bitwise Operator/1 -> counterGainIndex/1, fftCount/1
  Relational Operator1/1 -> Switch/2
  fftCount/1 -> Relational Operator/1
  fftValid/1 -> counterGainIndex/2, fftCount/2, Bitwise Operator/1
  Constant5/1 -> Relational Operator1/2, Relational Operator/2
  counterGainIndex/1 -> Switch/1, Relational Operator1/1
  Constant/1 -> Switch/3
  Switch/1 -> ROMindex/1

== system fftAnalysisSynthesis/fftAnalysisSynthesis/frequencyDomainProcessing/applyComplexGains/fftFilterCoefficients/filterChoice ==
  filterSelect : Inport
  ROMindex : Inport  Port=2
  Multiport Switch : MultiPortSwitch  DataPortOrder=Zero-based contiguous  Inputs=4  zeroidx=on  SaturateOnIntegerOverflow=off  InputSameDT=off
  filter1Coefficients : Subsystem
  filter2Coefficients : Subsystem
  filter3Coefficients : Subsystem
  filter4Coefficients : Subsystem
  filterCoefficients : Outport
  wires:
  Multiport Switch/1 -> filterCoefficients/1
  ROMindex/1 -> filter4Coefficients/1(ROMindex), filter3Coefficients/1(ROMindex), filter2Coefficients/1(ROMindex), filter1Coefficients/1(ROMindex)
  filter4Coefficients/1(complexCoefficients) -> Multiport Switch/5
  filter1Coefficients/1(complexCoefficients) -> Multiport Switch/2
  filter2Coefficients/1(complexCoefficients) -> Multiport Switch/3
  filterSelect/1 -> Multiport Switch/1
  filter3Coefficients/1(complexCoefficients) -> Multiport Switch/4

== system fftAnalysisSynthesis/fftAnalysisSynthesis/frequencyDomainProcessing/applyComplexGains/fftFilterCoefficients/filterChoice/filter1Coefficients ==
  ROMindex : Inport
  Real-Imag to Complex : RealImagToComplex
  filter1ImagCoefficients : Subsystem
  filter1RealCoefficients : Subsystem
  complexCoefficients : Outport
  wires:
  filter1ImagCoefficients/1(coefficentImag) -> Real-Imag to Complex/2
  ROMindex/1 -> filter1RealCoefficients/1(ROMindex), filter1ImagCoefficients/1(ROMindex)
  filter1RealCoefficients/1(coefficientReal) -> Real-Imag to Complex/1
  Real-Imag to Complex/1 -> complexCoefficients/1

== system fftAnalysisSynthesis/fftAnalysisSynthesis/frequencyDomainProcessing/applyComplexGains/fftFilterCoefficients/filterChoice/filter2Coefficients ==
  ROMindex : Inport
  Real-Imag to Complex : RealImagToComplex
  filter2ImagCoefficients : Subsystem
  filter2RealCoefficients : Subsystem
  complexCoefficients : Outport
  wires:
  filter2ImagCoefficients/1(coefficentImag) -> Real-Imag to Complex/2
  ROMindex/1 -> filter2RealCoefficients/1(ROMindex), filter2ImagCoefficients/1(ROMindex)
  filter2RealCoefficients/1(coefficientReal) -> Real-Imag to Complex/1
  Real-Imag to Complex/1 -> complexCoefficients/1

== system fftAnalysisSynthesis/fftAnalysisSynthesis/frequencyDomainProcessing/applyComplexGains/fftFilterCoefficients/filterChoice/filter3Coefficients ==
  ROMindex : Inport
  Real-Imag to Complex : RealImagToComplex
  filter3ImagCoefficients : Subsystem
  filter3RealCoefficients : Subsystem
  complexCoefficients : Outport
  wires:
  filter3ImagCoefficients/1(coefficentImag) -> Real-Imag to Complex/2
  ROMindex/1 -> filter3RealCoefficients/1(ROMindex), filter3ImagCoefficients/1(ROMindex)
  filter3RealCoefficients/1(coefficientReal) -> Real-Imag to Complex/1
  Real-Imag to Complex/1 -> complexCoefficients/1

== system fftAnalysisSynthesis/fftAnalysisSynthesis/frequencyDomainProcessing/applyComplexGains/fftFilterCoefficients/filterChoice/filter4Coefficients ==
  ROMindex : Inport
  Real-Imag to Complex : RealImagToComplex
  filter4ImagCoefficients : Subsystem
  filter4RealCoefficients : Subsystem
  complexCoefficients : Outport
  wires:
  filter4ImagCoefficients/1(coefficentImag) -> Real-Imag to Complex/2
  ROMindex/1 -> filter4RealCoefficients/1(ROMindex), filter4ImagCoefficients/1(ROMindex)
  filter4RealCoefficients/1(coefficientReal) -> Real-Imag to Complex/1
  Real-Imag to Complex/1 -> complexCoefficients/1

== system fftAnalysisSynthesis/fftAnalysisSynthesis/frequencyDomainProcessing/applyComplexGains/fftFilterCoefficients/filterChoice/filter1Coefficients/filter1ImagCoefficients ==
  ROMindex : Inport
  Lookup Table : Lookup_n-D  NumberOfTableDimensions=1  BreakpointsForDimension1=[0:modelParams.fft.size_half-1]  IndexSearchMethod=Evenly spaced points  Table=modelParams.fft_gains_1_imag  InterpMethod=Flat  ExtrapMethod=Clip  DiagnosticForOutOfRangeInput=Error  UseLastTableValue=on  OutDataTypeStr=modelParams.audio.dataType  RndMeth=Simplest
  Unit Delay : UnitDelay  SampleTime=-1  HasFrameUpgradeWarning=on
  coefficentImag : Outport  VectorParamsAs1DForOutWhenUnconnected=off
  wires:
  Unit Delay/1 -> coefficentImag/1
  ROMindex/1 -> Lookup Table/1
  Lookup Table/1 -> Unit Delay/1

== system fftAnalysisSynthesis/fftAnalysisSynthesis/frequencyDomainProcessing/applyComplexGains/fftFilterCoefficients/filterChoice/filter1Coefficients/filter1RealCoefficients ==
  ROMindex : Inport
  Lookup Table : Lookup_n-D  NumberOfTableDimensions=1  BreakpointsForDimension1=[0:modelParams.fft.size_half-1]  IndexSearchMethod=Evenly spaced points  Table=modelParams.fft_gains_1_real  InterpMethod=Flat  ExtrapMethod=Clip  DiagnosticForOutOfRangeInput=Error  UseLastTableValue=on  OutDataTypeStr=modelParams.audio.dataType  RndMeth=Simplest
  Unit Delay : UnitDelay  SampleTime=-1  HasFrameUpgradeWarning=on
  coefficientReal : Outport  VectorParamsAs1DForOutWhenUnconnected=off
  wires:
  Unit Delay/1 -> coefficientReal/1
  ROMindex/1 -> Lookup Table/1
  Lookup Table/1 -> Unit Delay/1

== system fftAnalysisSynthesis/fftAnalysisSynthesis/frequencyDomainProcessing/applyComplexGains/fftFilterCoefficients/filterChoice/filter2Coefficients/filter2ImagCoefficients ==
  ROMindex : Inport
  Lookup Table : Lookup_n-D  NumberOfTableDimensions=1  BreakpointsForDimension1=[0:modelParams.fft.size_half-1]  IndexSearchMethod=Evenly spaced points  Table=modelParams.fft_gains_2_imag  InterpMethod=Flat  ExtrapMethod=Clip  DiagnosticForOutOfRangeInput=Error  UseLastTableValue=on  OutDataTypeStr=modelParams.audio.dataType  RndMeth=Simplest
  Unit Delay : UnitDelay  SampleTime=-1  HasFrameUpgradeWarning=on
  coefficentImag : Outport  VectorParamsAs1DForOutWhenUnconnected=off
  wires:
  Unit Delay/1 -> coefficentImag/1
  ROMindex/1 -> Lookup Table/1
  Lookup Table/1 -> Unit Delay/1

== system fftAnalysisSynthesis/fftAnalysisSynthesis/frequencyDomainProcessing/applyComplexGains/fftFilterCoefficients/filterChoice/filter2Coefficients/filter2RealCoefficients ==
  ROMindex : Inport
  Lookup Table : Lookup_n-D  NumberOfTableDimensions=1  BreakpointsForDimension1=[0:modelParams.fft.size_half-1]  IndexSearchMethod=Evenly spaced points  Table=modelParams.fft_gains_2_real  InterpMethod=Flat  ExtrapMethod=Clip  DiagnosticForOutOfRangeInput=Error  UseLastTableValue=on  OutDataTypeStr=modelParams.audio.dataType  RndMeth=Simplest
  Unit Delay : UnitDelay  SampleTime=-1  HasFrameUpgradeWarning=on
  coefficientReal : Outport  VectorParamsAs1DForOutWhenUnconnected=off
  wires:
  Unit Delay/1 -> coefficientReal/1
  ROMindex/1 -> Lookup Table/1
  Lookup Table/1 -> Unit Delay/1

== system fftAnalysisSynthesis/fftAnalysisSynthesis/frequencyDomainProcessing/applyComplexGains/fftFilterCoefficients/filterChoice/filter3Coefficients/filter3ImagCoefficients ==
  ROMindex : Inport
  Lookup Table : Lookup_n-D  NumberOfTableDimensions=1  BreakpointsForDimension1=[0:modelParams.fft.size_half-1]  IndexSearchMethod=Evenly spaced points  Table=modelParams.fft_gains_3_imag  InterpMethod=Flat  ExtrapMethod=Clip  DiagnosticForOutOfRangeInput=Error  UseLastTableValue=on  OutDataTypeStr=modelParams.audio.dataType  RndMeth=Simplest
  Unit Delay : UnitDelay  SampleTime=-1  HasFrameUpgradeWarning=on
  coefficentImag : Outport  VectorParamsAs1DForOutWhenUnconnected=off
  wires:
  Unit Delay/1 -> coefficentImag/1
  ROMindex/1 -> Lookup Table/1
  Lookup Table/1 -> Unit Delay/1

== system fftAnalysisSynthesis/fftAnalysisSynthesis/frequencyDomainProcessing/applyComplexGains/fftFilterCoefficients/filterChoice/filter3Coefficients/filter3RealCoefficients ==
  ROMindex : Inport
  Lookup Table : Lookup_n-D  NumberOfTableDimensions=1  BreakpointsForDimension1=[0:modelParams.fft.size_half-1]  IndexSearchMethod=Evenly spaced points  Table=modelParams.fft_gains_3_real  InterpMethod=Flat  ExtrapMethod=Clip  DiagnosticForOutOfRangeInput=Error  UseLastTableValue=on  OutDataTypeStr=modelParams.audio.dataType  RndMeth=Simplest
  Unit Delay : UnitDelay  SampleTime=-1  HasFrameUpgradeWarning=on
  coefficientReal : Outport  VectorParamsAs1DForOutWhenUnconnected=off
  wires:
  Unit Delay/1 -> coefficientReal/1
  ROMindex/1 -> Lookup Table/1
  Lookup Table/1 -> Unit Delay/1

== system fftAnalysisSynthesis/fftAnalysisSynthesis/frequencyDomainProcessing/applyComplexGains/fftFilterCoefficients/filterChoice/filter4Coefficients/filter4ImagCoefficients ==
  ROMindex : Inport
  Lookup Table : Lookup_n-D  NumberOfTableDimensions=1  BreakpointsForDimension1=[0:modelParams.fft.size_half-1]  IndexSearchMethod=Evenly spaced points  Table=modelParams.fft_gains_4_imag  InterpMethod=Flat  ExtrapMethod=Clip  DiagnosticForOutOfRangeInput=Error  UseLastTableValue=on  OutDataTypeStr=modelParams.audio.dataType  RndMeth=Simplest
  Unit Delay : UnitDelay  SampleTime=-1  HasFrameUpgradeWarning=on
  coefficentImag : Outport  VectorParamsAs1DForOutWhenUnconnected=off
  wires:
  Unit Delay/1 -> coefficentImag/1
  ROMindex/1 -> Lookup Table/1
  Lookup Table/1 -> Unit Delay/1

== system fftAnalysisSynthesis/fftAnalysisSynthesis/frequencyDomainProcessing/applyComplexGains/fftFilterCoefficients/filterChoice/filter4Coefficients/filter4RealCoefficients ==
  ROMindex : Inport
  Lookup Table : Lookup_n-D  NumberOfTableDimensions=1  BreakpointsForDimension1=[0:modelParams.fft.size_half-1]  IndexSearchMethod=Evenly spaced points  Table=modelParams.fft_gains_4_real  InterpMethod=Flat  ExtrapMethod=Clip  DiagnosticForOutOfRangeInput=Error  UseLastTableValue=on  OutDataTypeStr=modelParams.audio.dataType  RndMeth=Simplest
  Unit Delay : UnitDelay  SampleTime=-1  HasFrameUpgradeWarning=on
  coefficientReal : Outport  VectorParamsAs1DForOutWhenUnconnected=off
  wires:
  Unit Delay/1 -> coefficientReal/1
  ROMindex/1 -> Lookup Table/1
  Lookup Table/1 -> Unit Delay/1

== matlab function fftAnalysisSynthesis/synthesis/OverlapAdd/fifo_state_machine2 ==
  data: valid input; pop output
function pop = fifo_state_machine(valid)
%#codegen

state_valid_low = fi(0, 0, 2, 0);
state_valid_high = fi(1, 0, 2, 0);
state_assert_pop = fi(2, 0, 2, 0);

persistent current_state;
if isempty(current_state)
    current_state = state_valid_low;
end

switch(current_state)
    case state_valid_low

        pop = false;
        
        if valid
            current_state = state_valid_high;
        else
            current_state = state_valid_low;
        end
        
    case state_valid_high
        
        pop = false;
        
        if valid
            current_state = state_valid_high;
        else
            current_state = state_assert_pop;
        end
        
    case state_assert_pop
        
        pop = true;
        
        current_state = state_assert_pop;
        
    otherwise
        
        pop = false;
        
end

== matlab function fftAnalysisSynthesis/synthesis/OverlapAdd/fifo_state_machine3 ==
  data: valid input; pop output
function pop = fifo_state_machine(valid)
%#codegen

state_valid_low = fi(0, 0, 2, 0);
state_valid_high = fi(1, 0, 2, 0);
state_assert_pop = fi(2, 0, 2, 0);

persistent current_state;
if isempty(current_state)
    current_state = state_valid_low;
end

switch(current_state)
    case state_valid_low

        pop = false;
        
        if valid
            current_state = state_valid_high;
        else
            current_state = state_valid_low;
        end
        
    case state_valid_high
        
        pop = false;
        
        if valid
            current_state = state_valid_high;
        else
            current_state = state_assert_pop;
        end
        
    case state_assert_pop
        
        pop = true;
        
        current_state = state_assert_pop;
        
    otherwise
        
        pop = false;
        
end

== matlab function fftAnalysisSynthesis/synthesis/OverlapAdd/fifo_state_machine4 ==
  data: valid input; pop output
function pop = fifo_state_machine(valid)
%#codegen

state_valid_low = fi(0, 0, 2, 0);
state_valid_high = fi(1, 0, 2, 0);
state_assert_pop = fi(2, 0, 2, 0);

persistent current_state;
if isempty(current_state)
    current_state = state_valid_low;
end

switch(current_state)
    case state_valid_low

        pop = false;
        
        if valid
            current_state = state_valid_high;
        else
            current_state = state_valid_low;
        end
        
    case state_valid_high
        
        pop = false;
        
        if valid
            current_state = state_valid_high;
        else
            current_state = state_assert_pop;
        end
        
    case state_assert_pop
        
        pop = true;
        
        current_state = state_assert_pop;
        
    otherwise
        
        pop = false;
        
end

== matlab function fftAnalysisSynthesis/synthesis/OverlapAdd/fifoWriteSelect ==
  data: fifo_counter input; valid_1 output; valid_signal input; valid_2 output; valid_3 output; valid_4 output
function [valid_1, valid_2, valid_3, valid_4] = fifoSelect(fifo_counter, valid_signal)
%#codegen



switch fifo_counter
    case 0
        valid_1 = valid_signal;
        valid_2 = false;
        valid_3 = false;
        valid_4 = false;
    case 1
        valid_1 = false;
        valid_2 = valid_signal;
        valid_3 = false;
        valid_4 = false;
    case 2
        valid_1 = false;
        valid_2 = false;
        valid_3 = valid_signal;
        valid_4 = false;
    case 3
        valid_1 = false;
        valid_2 = false;
        valid_3 = false;
        valid_4 = valid_signal;
    otherwise
        valid_1 = false;
        valid_2 = false;
        valid_3 = false;
        valid_4 = false;
       
end

== matlab function fftAnalysisSynthesis/synthesis/OverlapAdd/fifo_state_machine1 ==
  data: valid input; pop output
function pop = fifo_state_machine(valid)
%#codegen

state_valid_low  = fi(0, 0, 2, 0);
state_valid_high = fi(1, 0, 2, 0);
state_assert_pop = fi(2, 0, 2, 0);

persistent current_state;
if isempty(current_state)
    current_state = state_valid_low;
end

switch(current_state)
    case state_valid_low

        pop = false;
        
        if valid
            current_state = state_valid_high;
        else
            current_state = state_valid_low;
        end
        
    case state_valid_high
        
        pop = false;
        
        if valid
            current_state = state_valid_high;
        else
            current_state = state_assert_pop;
        end
        
    case state_assert_pop
        
        pop = true;
        
        current_state = state_assert_pop;
        
    otherwise
        
        pop = false;
        
end
